simulink model "Inverse_dynamic_controller"  (R2019b)
settings: Solver=ode4  StartTime=0.0  StopTime=50  FixedStep=0.01  RelTol=1e-3
settings Model: Creator=USER  LastModifiedBy=USER

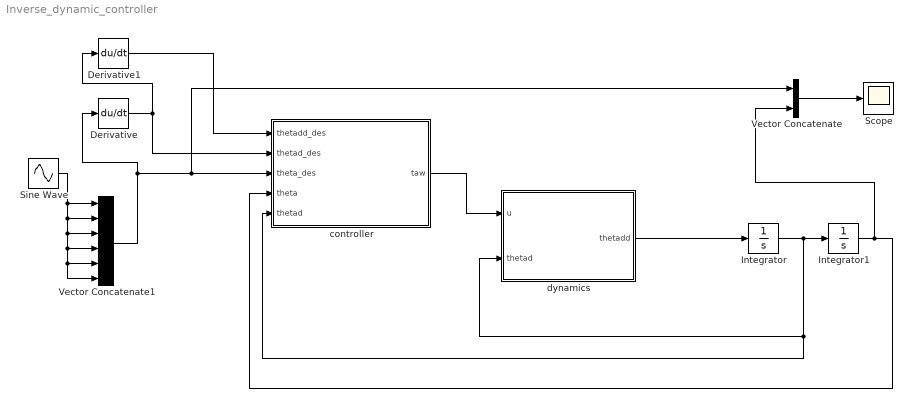
== system Inverse_dynamic_controller ==
  Derivative : Derivative
  Derivative1 : Derivative
  Integrator : Integrator  InitialCondition=[0.1;0.1;0.1;0.1;0.1;0.1]
  Integrator1 : Integrator  InitialCondition=[0.1;0.1;0.1;0.1;0.1;0.1]
  Scope : Scope
  Sine Wave : Sin  Bias=2  SampleTime=0
  Vector Concatenate : Concatenate
  Vector Concatenate1 : Concatenate  NumInputs=6
  controller : MATLAB Function  TreatAsAtomicUnit=on
  dynamics : MATLAB Function  TreatAsAtomicUnit=on
  wires:
  dynamics/1(thetadd) -> Integrator/1
  Integrator/1 -> dynamics/2(thetad), controller/5(thetad), Integrator1/1
  Integrator1/1 -> Vector Concatenate/2, controller/4(theta)
  controller/1(taw) -> dynamics/1(u)
  Vector Concatenate/1 -> Scope/1
  Sine Wave/1 -> Vector Concatenate1/1, Vector Concatenate1/3, Vector Concatenate1/6, Vector Concatenate1/5, Vector Concatenate1/4, Vector Concatenate1/2
  Vector Concatenate1/1 -> Vector Concatenate/1, controller/3(theta_des), Derivative/1
  Derivative/1 -> Derivative1/1, controller/2(thetad_des)
  Derivative1/1 -> controller/1(thetadd_des)

== matlab function Inverse_dynamic_controller/controller ==
  data: thetadd_des input; taw output; thetad_des input; theta_des input; theta input; thetad input
function taw = fcn(thetadd_des,thetad_des,theta_des,theta,thetad)
G=[                125/576460752303423488;
        6243369967885135/2199023255552;
        1843278687284175/4398046511104;
 -7769952016327311/1152921504606846976;
     2257351121598699/2251799813685248;
                                     0.1];
M=[ 52.4722   -0.0003    0.0028   -0.0503   -0.0001    0.0000;
  104.8982  290.5285  163.8569   85.7264   85.2726   85.2667;
   85.2667  115.8130  148.4693   85.6721   85.2726   85.2667;
   -0.0119   -0.0070   -0.0097   -0.0017   -0.0067   -0.0067;
    0.6575    0.7170    0.9633    0.6800    0.6687    0.6627;
         0.1         0.1         0.1         0.1         0.1         0.1]
C=[261.8493         0         0   -0.0005         0         0;
   -4.1701   76.1836   58.8031    0.3261   -0.0000   -0.0000;
  -60.4552   -6.5177    2.5168    0.0520    0.0000    0.0000;
   -0.0055         0         0    0.0005         0         0;
   -0.4221   -0.0217   -0.0460   -0.3403         0         0;
         0.1         0.1         0.1         0.1         0.1         0.1]

e=theta_des-theta
edot=-thetad
Kp=[10 0 0 0 0 0;0 20 0 0 0 0;0 0 30 0 0 0;0 0 0 40 0 0;0 0 0 0 50 0;0 0 0 0 0 60]
Kd=[2 0 0 0 0 0;0 4 0 0 0 0;0 0 6 0 0 0;0 0 0 8 0 0;0 0 0 0 10 0;0 0 0 0 0 12]
taw=M*(thetadd_des+Kd*edot+Kp*e)+C*thetad+G

== matlab function Inverse_dynamic_controller/dynamics ==
  data: u input; thetadd output; thetad input
function thetadd = fcn(u,thetad)
G=[                125/576460752303423488;
        6243369967885135/2199023255552;
        1843278687284175/4398046511104;
 -7769952016327311/1152921504606846976;
     2257351121598699/2251799813685248;
                                    0.1];
M=[ 52.4722   -0.0003    0.0028   -0.0503   -0.0001    0.0000;
  104.8982  290.5285  163.8569   85.7264   85.2726   85.2667;
   85.2667  115.8130  148.4693   85.6721   85.2726   85.2667;
   -0.0119   -0.0070   -0.0097   -0.0017   -0.0067   -0.0067;
    0.6575    0.7170    0.9633    0.6800    0.6687    0.6627;
         0.1         .10         .10         .10         .10         .10]
C=[261.8493         0         0   -0.0005         0         0;
   -4.1701   76.1836   58.8031    0.3261   -0.0000   -0.0000;
  -60.4552   -6.5177    2.5168    0.0520    0.0000    0.0000;
   -0.0055         0         0    0.0005         0         0;
   -0.4221   -0.0217   -0.0460   -0.3403         0         0;
         .10         .10         .10         .10         .10         .10]
     thetadd=inv(M)*(u-C*thetad-G);
